simulink model "Observer_particle_dist"  (R2017a)
settings: Solver=FixedStepAuto  StartTime=0.0  StopTime=6  FixedStep=0.0001  RelTol=1e-3  EnableMultiTasking=on
settings Model: Creator=DR_C  LastModifiedBy=Merc
settings DataIOCC: LimitDataPoints=on
settings OptimizationCC: LifeSpan=inf
settings DebuggingCC: AllowSymbolicDim=off  SFUnexpectedBacktrackingDiag=warning  SFNoUnconditionalDefaultTransitionDiag=warning  SFExecutionAtInitializationDiag=none
settings ModelReferenceCC: PropagateSignalLabelsOutOfModel=off
settings GRTTargetCC: TargetLangStandard=C89/C90 (ANSI)
settings ConfigComp: CovMetricSettings=dw  CovHtmlReporting=on  CovSaveCumulativeToWorkspaceVar=on  CovSaveSingleToWorkspaceVar=on  CovExternalEMLEnable=off

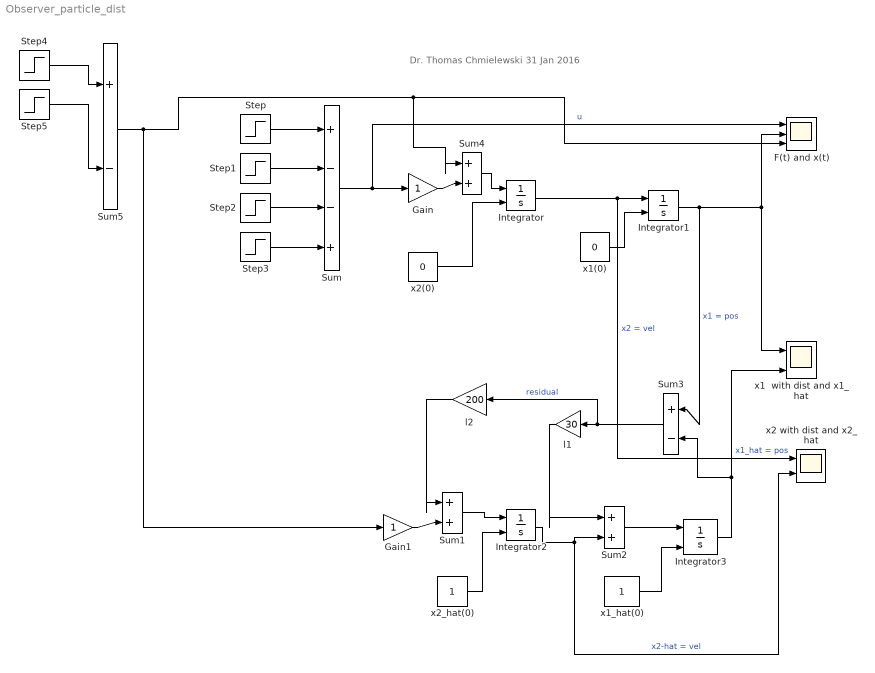
== system Observer_particle_dist ==
  note: Dr. Thomas Chmielewski 31 Jan 2016
  F(t) and x(t) : Scope  NumInputPorts=3
  Gain : Gain
  Gain1 : Gain
  Integrator{,1..3} (4 alike) : Integrator  InitialConditionSource=external
  Step : Step  Time=0  SampleTime=0
  Step1 : Step  SampleTime=0
  Step2 : Step  Time=3  SampleTime=0
  Step3 : Step  Time=4  SampleTime=0
  Step4 : Step  Time=3.25  SampleTime=0
  Step5 : Step  Time=3.5  SampleTime=0
  Sum : Sum  Inputs=+--+
  Sum1 : Sum  Inputs=|++
  Sum2 : Sum  Inputs=|++
  Sum3 : Sum  Inputs=|+-
  Sum4 : Sum  Inputs=|++
  Sum5 : Sum  Inputs=+-
  l1 : Gain  Gain=30
  l2 : Gain  Gain=200
  x1  with dist and x1_hat : Scope  NumInputPorts=2
  x1(0) : Constant  Value=0
  x1_hat(0) : Constant
  x2 with dist and x2_hat : Scope  NumInputPorts=2
  x2(0) : Constant  Value=0
  x2_hat(0) : Constant
  wires:
  Sum/1 -> Gain/1, F(t) and x(t)/1  "u"
  Step3/1 -> Sum/4
  Step2/1 -> Sum/3
  Step1/1 -> Sum/2
  Step/1 -> Sum/1
  Integrator1/1 -> Sum3/1, x1  with dist and x1_hat/1, F(t) and x(t)/2  "x1 = pos"
  x2(0)/1 -> Integrator/2
  x1(0)/1 -> Integrator1/2
  Integrator3/1 -> x1  with dist and x1_hat/2, Sum3/2  "x1_hat = pos"
  x2_hat(0)/1 -> Integrator2/2
  x1_hat(0)/1 -> Integrator3/2
  Gain1/1 -> Sum1/2
  Sum1/1 -> Integrator2/1
  Sum2/1 -> Integrator3/1
  Integrator2/1 -> x2 with dist and x2_hat/2, Sum2/2  "x2-hat = vel"
  l1/1 -> Sum2/1
  l2/1 -> Sum1/1
  Sum3/1 -> l2/1, l1/1  "residual"
  Integrator/1 -> x2 with dist and x2_hat/1, Integrator1/1  "x2 = vel"
  Step5/1 -> Sum5/2
  Step4/1 -> Sum5/1
  Sum5/1 -> Gain1/1, Sum4/1, F(t) and x(t)/3
  Gain/1 -> Sum4/2
  Sum4/1 -> Integrator/1
